simulink model "fourier_example"  (R2021b)
settings: Solver=FixedStepDiscrete  StartTime=0.0  StopTime=0.1  FixedStep=1/100000  MaxStep=10/1000  RelTol=1e-3  EnableMultiTasking=on
libraries: dspspect3 x1
settings Model: Creator=eg572583  LastModifiedBy=eechris
settings SolverCC: AlgebraicLoopSolver=TrustRegion
settings DataIOCC: LimitDataPoints=on  SaveFormat=Array  SignalLoggingSaveFormat=ModelDataLogs  ReturnWorkspaceOutputs=off
settings OptimizationCC: LifeSpan=inf
settings DebuggingCC: UnderspecifiedInitializationDetection=Classic  MergeDetectMultiDrivingBlocksExec=none  SolverPrmCheckMsg=warning  MultiTaskDSMMsg=warning  MultiTaskCondExecSysMsg=none  SFUnexpectedBacktrackingDiag=warning  SFNoUnconditionalDefaultTransitionDiag=warning  SFExecutionAtInitializationDiag=none  SFMachineParentedDataDiag=warning  ArithmeticOperatorsInVariantConditions=warning
settings HardwareCC: ProdBitPerPointer=32  ProdBitPerSizeT=32  ProdBitPerPtrDiffT=32  ProdLargestAtomicFloat=None  ProdIntDivRoundTo=Undefined  ProdEndianess=Unspecified  ProdWordSize=32  ProdHWDeviceType=32-bit Generic
settings ModelReferenceCC: PropagateSignalLabelsOutOfModel=off
settings SFSimCC: SimUseLocalCustomCode=off  CustomCodeUndefinedFunction=UseInterfaceOnly
settings RTWCC: RTWUseLocalCustomCode=off
settings CodeAppCC: StateflowObjectComments=on
settings GRTTargetCC: TargetLangStandard=C89/C90 (ANSI)
settings ConfigComp: CovMetricSettings=dw  CovSaveCumulativeToWorkspaceVar=on  CovSaveSingleToWorkspaceVar=on  CovExternalEMLEnable=off

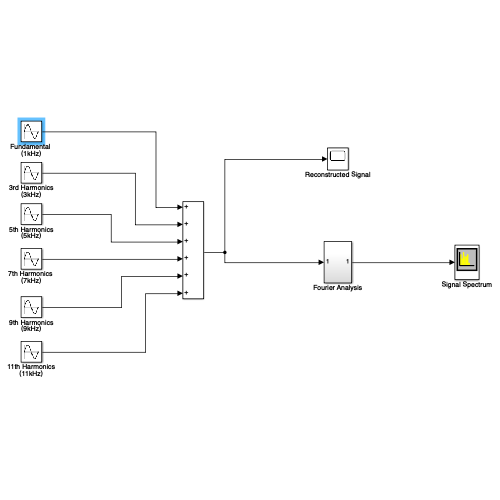
[thumbnail: Simulink's stored preview of the top-level diagram]
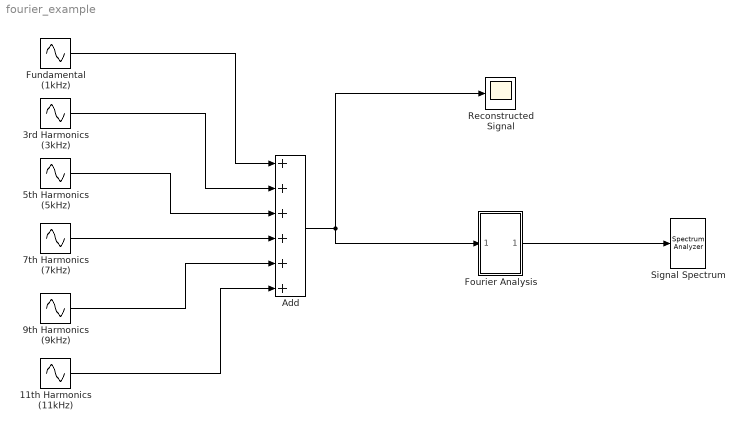
== system fourier_example ==
  11th Harmonics (11kHz) : Sin  Amplitude=0.1157  Frequency=11000*2*pi  SampleTime=0
  3rd Harmonics (3kHz) : Sin  Amplitude=0.4244  Frequency=3*1000*2*pi  SampleTime=0
  5th Harmonics (5kHz) : Sin  Amplitude=0.2546  Frequency=5000*2*pi  SampleTime=0
  7th Harmonics (7kHz) : Sin  Amplitude=0.1819  Frequency=7000*2*pi  SampleTime=0
  9th Harmonics (9kHz) : Sin  Amplitude=0.1415  Frequency=9000*2*pi  SampleTime=0
  Add : Sum  Inputs=++++++
  Fourier Analysis : Subsystem
  Fundamental (1kHz) : Sin  Amplitude=1.273  Frequency=1000*2*pi  SampleTime=0
  Reconstructed Signal : Scope
  Signal Spectrum : SpectrumAnalyzer
  wires:
  Fundamental (1kHz)/1 -> Add/1
  3rd Harmonics (3kHz)/1 -> Add/2
  5th Harmonics (5kHz)/1 -> Add/3
  7th Harmonics (7kHz)/1 -> Add/4
  9th Harmonics (9kHz)/1 -> Add/5
  11th Harmonics (11kHz)/1 -> Add/6
  Add/1 -> Fourier Analysis/1(In1), Reconstructed Signal/1
  Fourier Analysis/1(Out1) -> Signal Spectrum/1

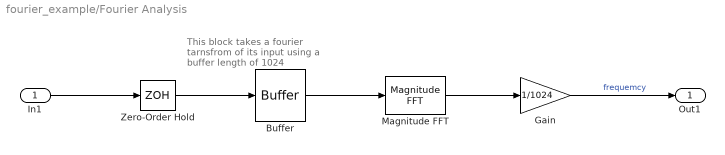
== system fourier_example/Fourier Analysis ==
  note: This block takes a fourier tarnsfrom of its input using a buffer length of 1024
  In1 : Inport
  Buffer : Buffer  N=1024
  Gain : Gain  Gain=1/1024
  Magnitude FFT : dspspect3/Magnitude FFT  mag_or_magsq=Magnitude  FFTImplementation=Auto  fftLenInherit=off  fftsize=1024  WrapInput=on
      settings: SourceProductBaseCode=DS
  Zero-Order Hold : ZeroOrderHold  SampleTime=50e-6
  Out1 : Outport
  wires:
  Magnitude FFT/1 -> Gain/1
  Gain/1 -> Out1/1  "frequemcy"
  In1/1 -> Zero-Order Hold/1
  Zero-Order Hold/1 -> Buffer/1
  Buffer/1 -> Magnitude FFT/1
